simulink model "fc_KTH_lib"  (Simulink 4.00)
settings: Solver=FixedStepDiscrete  StartTime=0.0  StopTime=5  RelTol=1e-3
undefined symbols (not defined in the file or in its folder): cell_const_F, cell_const_g, cell_const_jo, cell_const_LHV_H2, cell_const_Mair, cell_const_MH, cell_const_MW, cell_const_R2, cell_const_Voc, fan_cool, fc_act, fc_blower_rec_H2, fc_blowera, fc_cell_const_eta1, fc_cell_const_eta_DCDC, fc_cell_const_etablow, fc_cell_const_etagen, fc_cell_const_etapump, fc_cell_const_ex, fc_cell_const_kw, fc_cell_const_Nrad, fc_cell_const_U, fc_cell_dim_A, fc_cell_dim_tm, fc_cell_press_a, fc_cell_press_amb, fc_cell_press_an, fc_cell_press_blowa, fc_cell_press_blowr, fc_cell_press_c, fc_cell_press_hum, fc_cell_press_hyd, fc_cell_stack_dpipe, fc_cell_stack_dpipefc, fc_cell_stack_drad, fc_cell_stack_Lpipe, fc_cell_stack_Lpipefc, fc_cell_stack_Lrad, fc_cell_stack_N, fc_cell_stack_Pel, fc_cell_stoich_RHah, fc_cell_stoich_RHch, fc_cell_stoich_RHo, fc_cell_stoich_vH, fc_cell_stoich_vO, fc_cell_stoich_XON, fc_cell_temp_ah, fc_cell_temp_amb, fc_cell_temp_cell, fc_cell_temp_ch, fc_cell_temp_cond, fc_cell_temp_cool, fc_cell_temp_evap, fc_cell_temp_rad, fc_cell_temp_ref, fc_compressor, fc_conda, fc_condc, fc_coolstack, fc_current ... (+10)
(part 1 of 2)
settings Model: LastModifiedBy=kharalds

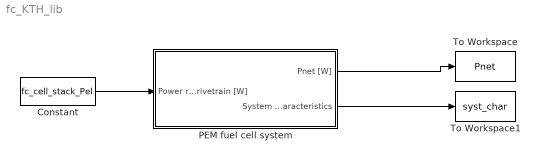
== system fc_KTH_lib ==
  Constant : Constant  Value=fc_cell_stack_Pel
  PEM fuel cell system : Subsystem
      settings: RTWFcnNameOpts=Auto  RTWFileNameOpts=Auto
  To Workspace : ToWorkspace  VariableName=Pnet  SampleTime=-1  SaveFormat=Array
  To Workspace1 : ToWorkspace  VariableName=syst_char  SampleTime=-1  SaveFormat=Array
  wires:
  Constant/1 -> PEM fuel cell system/1("Power request from drivetrain [W] ")
  PEM fuel cell system/1(Pnet [W]) -> To Workspace/1
  PEM fuel cell system/2(System characteristics) -> To Workspace1/1

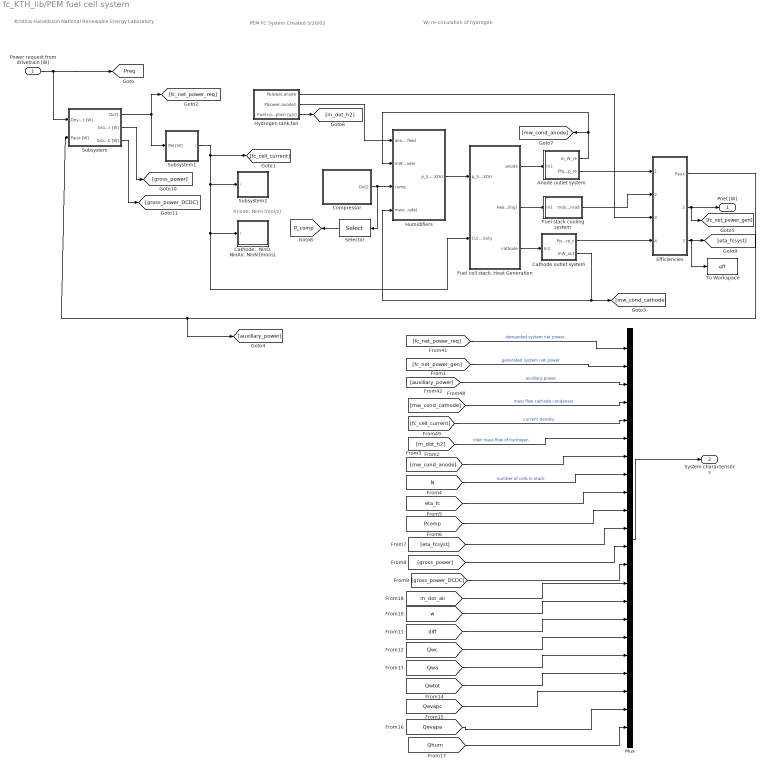
== system fc_KTH_lib/PEM fuel cell system ==
  note: Kristina Haraldsson
      | National Renewable Energy Laboratory
  note: PEM FC System
      | Created  3/20/02
  note: W/ re-circulation of hydrogen
  note: Anode: NinH [mol/s]
  "Power request from drivetrain [W] " : Inport  Port=1  LatchInput=off
  Anode outlet system : Subsystem
      settings: RTWFcnNameOpts=Auto  RTWFileNameOpts=Auto
  Cathode outlet system : Subsystem
      settings: RTWFcnNameOpts=Auto  RTWFileNameOpts=Auto
  "Cathode:  NinO, NinAir, NinN [mol/s]" : Subsystem
      settings: RTWFcnNameOpts=Auto  RTWFileNameOpts=Auto
  "Compressor " : Subsystem
      settings: RTWFcnNameOpts=Auto  RTWFileNameOpts=Auto
  Efficiencies : Subsystem
      settings: RTWFcnNameOpts=Auto  RTWFileNameOpts=Auto
  "Fuel cell stack, Heat Generation" : Subsystem
      settings: RTWFcnNameOpts=Auto  RTWFileNameOpts=Auto
  Fuel stack cooling system : Subsystem
      settings: RTWFcnNameOpts=Auto  RTWFileNameOpts=Auto
  Humidifiers : Subsystem
      settings: RTWFcnNameOpts=Auto  RTWFileNameOpts=Auto
  Hydrogen tank,fan : Subsystem
      settings: RTWFcnNameOpts=Auto  RTWFileNameOpts=Auto
  Mux : Mux  Inputs=22
  Selector : Selector  Orientation=left  InputType=Vector  ElementSrc=Internal  Elements=[4]  RowSrc=Internal  Rows=1  ColumnSrc=Internal  Columns=1  InputPortWidth=7
  Subsystem : Subsystem
      settings: RTWFcnNameOpts=Auto  RTWFileNameOpts=Auto
  Subsystem1 : Subsystem
      settings: RTWFcnNameOpts=Auto  RTWFileNameOpts=Auto
  Subsystem2 : Subsystem
      settings: RTWFcnNameOpts=Auto  RTWFileNameOpts=Auto
  To Workspace : ToWorkspace  VariableName=eff  SampleTime=-1  SaveFormat=Array
  Pnet [W] : Outport  Port=1
  System characteristics : Outport  Port=2
  tag scope: P_comp=global, Preq=global
  wires:
  Humidifiers/1("p_56 anode feed p_57 cathode feed Psat Psatah Psatch XWaI,  XWcI  XOcI ") -> "Fuel cell stack, Heat Generation"/1("p_56, NinH, p_57, NinAir, Psat,Psatah,PsatchXWaI, XWcI, XOcI")
  "Compressor "/1(Out2) -> Humidifiers/3(comp), Selector/1
  "Fuel cell stack, Heat Generation"/1(anode) -> Anode outlet system/1(In1)
  "Fuel cell stack, Heat Generation"/2(Heat_fc (fuel cell stack cooling)) -> Fuel stack cooling system/1(In1)
  Fuel stack cooling system/1(mdotW P_pump A Heat Qcool P_fanrad) -> Efficiencies/2(P_pump,cool P_fanrad)
  Anode outlet system/2(Pfan Ppump_re) -> Efficiencies/1("P_fan_,re, P_pump_re_a")
  Anode outlet system/1(m_W_re) -> Humidifiers/2(mW_out(anode)), [mw_cond_anode]
  "Fuel cell stack, Heat Generation"/3(cathode) -> Cathode outlet system/1(In1)
  Cathode outlet system/1(Ppump_re_c) -> Efficiencies/4(P_pump_re_c)
  Cathode outlet system/2(mW_out) -> Humidifiers/4(mwout(cathode)), [mw_cond_cathode]
  Hydrogen tank,fan/1(Pblower,anode) -> Efficiencies/3(P_fan,anode)
  Efficiencies/1(Paux) -> Subsystem/2(Paux [W]), [auxiliary_power]
  Subsystem/1(Out1) -> Subsystem1/1(Pel [W]), [fc_net_power_req]
  "Power request from drivetrain [W] "/1 -> Subsystem/1(Drivetrain Power Request [W]), [Preq]
  Subsystem1/1(i) -> Subsystem2/1(i), "Cathode:  NinO, NinAir, NinN [mol/s]"/1(i), "Fuel cell stack, Heat Generation"/2(Current density), [fc_cell_current]
  Hydrogen tank,fan/3(Fuel consumption [g/s]) -> [m_dot_h2]
  Hydrogen tank,fan/2(Pblower,anode1) -> Humidifiers/1(anode feed)
  [fc_net_power_req] -> Mux/1  "demanded system net power"
  [auxiliary_power] -> Mux/3  "auxiliary power"
  [mw_cond_cathode] -> Mux/4  "mass flow cathode condenser"
  [fc_cell_current] -> Mux/5  "current density"
  [fc_net_power_gen] -> Mux/2  "generated system net power"
  Mux/1 -> System characteristics/1
  [m_dot_h2] -> Mux/6  "inlet mass flow of hydrogen"
  [mw_cond_anode] -> Mux/7
  [N] -> Mux/8  "number of cells in stack"
  [eta_fc] -> Mux/9
  [Pcomp] -> Mux/10
  Selector/1 -> [P_comp]
  Subsystem/2(Gross power [W]) -> [gross_power]
  Efficiencies/2(Pnet [W]) -> Pnet [W]/1, [fc_net_power_gen]
  Efficiencies/3(eta_fcsyst) -> [eta_fcsyst], To Workspace/1
  Subsystem/3(Gross power incl. DCDC [W]) -> [gross_power_DCDC]
  [eta_fcsyst] -> Mux/11
  [gross_power] -> Mux/12
  [gross_power_DCDC] -> Mux/13
  [Qhum] -> Mux/22
  [Qevapa] -> Mux/21
  [Qevapc] -> Mux/20
  [Qwtot] -> Mux/19
  [Qwa] -> Mux/18
  [Qwc] -> Mux/17
  [diff] -> Mux/16
  [w] -> Mux/15
  [m_dot_air] -> Mux/14

== system fc_KTH_lib/PEM fuel cell system/Anode outlet system ==
  note: Anode outlet system
  In1 : Inport  Port=1  LatchInput=off
  Anode condenser : Subsystem
      settings: RTWFcnNameOpts=Auto  RTWFileNameOpts=Auto
  Mux : Mux  Inputs=2
  Mux1 : Mux  Inputs=2
  "Re-circulation: Blower_rec, pump" : Subsystem
      settings: RTWFcnNameOpts=Auto  RTWFileNameOpts=Auto
  Vent/Purge : Subsystem
      settings: RTWFcnNameOpts=Auto  RTWFileNameOpts=Auto
  m_W_re : Outport  Port=1
  Pfan Ppump_re : Outport  Port=2
  tag scope: NoutH=global
  wires:
  In1/1 -> Anode condenser/1(In1)
  Anode condenser/1(Out1) -> Vent/Purge/1(In1)
  Vent/Purge/1(Out1) -> "Re-circulation: Blower_rec, pump"/1(In1)
  "Re-circulation: Blower_rec, pump"/3(p_70) -> Mux/2
  "Re-circulation: Blower_rec, pump"/4(Pfan) -> Mux1/1
  "Re-circulation: Blower_rec, pump"/5(Ppump_re) -> Mux1/2
  Mux1/1 -> Pfan Ppump_re/1
  "Re-circulation: Blower_rec, pump"/1(m_W_re) -> m_W_re/1
  "Re-circulation: Blower_rec, pump"/2(NoutH_re) -> Mux/1
  Mux/1 -> [NoutH]

== system fc_KTH_lib/PEM fuel cell system/Cathode outlet system ==
  note: Cathode outlet system
  In1 : Inport  Port=1  LatchInput=off
  Cathode condenser : Subsystem
      settings: RTWFcnNameOpts=Auto  RTWFileNameOpts=Auto
  Pump (cathode) : Subsystem
      settings: RTWFcnNameOpts=Auto  RTWFileNameOpts=Auto
  Ppump_re_c : Outport  Port=1
  mW_out : Outport  Port=2
  wires:
  In1/1 -> Cathode condenser/1(In1)
  Pump (cathode)/1(Ppump_re_c) -> Ppump_re_c/1
  Cathode condenser/1(mw_out1) -> Pump (cathode)/1(In1)
  Pump (cathode)/2(mW_out) -> mW_out/1

== system fc_KTH_lib/PEM fuel cell system/Cathode:  NinO, NinAir, NinN [mol/s] ==
  note: Total cathode molar flow
  i : Inport  Port=1  LatchInput=off
  Constant : Constant  Value=fc_cell_stoich_vO
  Constant1 : Constant  Value=fc_cell_dim_A
  Constant2 : Constant  Value=fc_cell_stack_N
  Constant3 : Constant  Value=cell_const_F
  Constant4 : Constant  Value=4
  Constant5 : Constant  Value=fc_cell_stoich_XON
  Constant6 : Constant  Value=fc_cell_stoich_XON
  Constant7 : Constant  Value=1
  Constant8 : Constant  Value=cell_const_Mair
  Product : Product  Inputs=4  Multiplication=Element-wise(.*)  SaturateOnIntegerOverflow=on
  Product1 : Product  Inputs=*/  Multiplication=Element-wise(.*)  SaturateOnIntegerOverflow=on
  Product2 : Product  Inputs=2  Multiplication=Element-wise(.*)  SaturateOnIntegerOverflow=on
  Product3 : Product  Inputs=*/  Multiplication=Element-wise(.*)  SaturateOnIntegerOverflow=on
  Product4 : Product  Inputs=2  Multiplication=Element-wise(.*)  SaturateOnIntegerOverflow=on
  Product5 : Product  Inputs=2  Multiplication=Element-wise(.*)  SaturateOnIntegerOverflow=on
  Sum : Sum  Inputs=|+-  SaturateOnIntegerOverflow=on
  tag scope: NinAir=global, NinN=global, NinO=global, m_dot_air=global
  wires:
  Constant1/1 -> Product/3
  Constant/1 -> Product/2
  i/1 -> Product/1
  Constant2/1 -> Product/4
  Product/1 -> Product1/1
  Constant4/1 -> Product2/2
  Product2/1 -> Product1/2
  Product1/1 -> Product3/1, [NinO]
  Constant5/1 -> Product3/2
  Product3/1 -> Product4/1, Product5/1, [NinAir]
  Constant7/1 -> Sum/1
  Constant6/1 -> Sum/2
  Sum/1 -> Product4/2
  Product4/1 -> [NinN]
  Constant3/1 -> Product2/1
  Constant8/1 -> Product5/2
  Product5/1 -> [m_dot_air]

== system fc_KTH_lib/PEM fuel cell system/Compressor  ==
  note: Compressor
  Cathode pressure : Constant  Value=fc_cell_press_c
  "Initial value, 0.1 mole/s" : Memory  X0=0.1  InheritSampleTime=off
      settings: RTWStateStorageClass=Auto
  M_air [g/mol] : Constant  Value=cell_const_Mair
  Mass flow [g/s]  discharge pressure [bar(a)] CompOA1050 (Opcon) : Lookup  InputValues=[Qm_1050]  OutputValues=[p2_1050]
  Mass flow [g/s] Pcomp [W] CompOA1050 (Opcon) : Lookup  InputValues=[Qm_1050]  OutputValues=[Pcomp_1050]
  Mass flow [g/s] discharge temperature [C] CompOA1050 (Opcon)1 : Lookup  InputValues=[Qm_1050]  OutputValues=[T2_1050]
  Mux : Mux  Inputs=5
  Product : Product  Inputs=2  Multiplication=Element-wise(.*)  SaturateOnIntegerOverflow=on
  fc_compressor.m : MATLABFcn  MATLABFcn=fc_compressor(u,fc_cell_press_amb,fc_cell_temp_amb,fc_cell_const_eta1,fc_cell_const_etagen,fc_cell_stoich_RHo,fc_cell_press_hum,fc_cell_temp_evap,fc_cell_temp_cell,fc_cell_stack_Pel)  OutputDimensions=7  OutputSignalType=auto  Output1D=on
  Out2 : Outport  Port=1
  wires:
  M_air [g/mol]/1 -> Product/2
  Mux/1 -> fc_compressor.m/1
  fc_compressor.m/1 -> Out2/1
  Mass flow [g/s]  discharge pressure [bar(a)] CompOA1050 (Opcon)/1 -> Mux/2
  Mass flow [g/s] Pcomp [W] CompOA1050 (Opcon)/1 -> Mux/3
  [NinAir] -> "Initial value, 0.1 mole/s"/1
  "Initial value, 0.1 mole/s"/1 -> Mux/1, Product/1
  Product/1 -> Mass flow [g/s]  discharge pressure [bar(a)] CompOA1050 (Opcon)/1, Mass flow [g/s] Pcomp [W] CompOA1050 (Opcon)/1, Mass flow [g/s] discharge temperature [C] CompOA1050 (Opcon)1/1
  Mass flow [g/s] discharge temperature [C] CompOA1050 (Opcon)1/1 -> Mux/4
  Cathode pressure/1 -> Mux/5

== system fc_KTH_lib/PEM fuel cell system/Efficiencies ==
  note: Efficiencies
  "P_fan_,re, P_pump_re_a" : Inport  Port=1  LatchInput=off
  P_pump,cool P_fanrad : Inport  Port=2  LatchInput=off
  P_fan,anode : Inport  Port=3  LatchInput=off
  P_pump_re_c : Inport  Port=4  LatchInput=off
  Constant : Constant  Value=cell_const_LHV_H2
  Demux : Demux  Outputs=2  BusSelectionMode=off
  Demux1 : Demux  Outputs=2  BusSelectionMode=off
  Product : Product  Inputs=*/  Multiplication=Element-wise(.*)  SaturateOnIntegerOverflow=on
  Product1 : Product  Inputs=2  Multiplication=Element-wise(.*)  SaturateOnIntegerOverflow=on
  Selector1 : Selector  InputType=Vector  ElementSrc=Internal  Elements=[2 6]  RowSrc=Internal  Rows=1  ColumnSrc=Internal  Columns=1  InputPortWidth=6
  Sum{,1..6} (7 alike) : Sum  Inputs=|++  SaturateOnIntegerOverflow=on
  Sum7 : Sum  Inputs=|-+  SaturateOnIntegerOverflow=on
  Paux : Outport  Port=1
  Pnet [W] : Outport  Port=2
  eta_fcsyst : Outport  Port=3
  tag scope: Pcomp=global
  wires:
  P_pump,cool P_fanrad/1 -> Selector1/1
  [P_comp] -> Sum/1, [Pcomp]
  "P_fan_,re, P_pump_re_a"/1 -> Demux/1
  P_pump_re_c/1 -> Sum6/2
  P_fan,anode/1 -> Sum5/2
  Demux/1 -> Sum3/2
  Demux/2 -> Sum4/2
  [P_fancool] -> Sum/2
  Sum/1 -> Sum1/1
  Selector1/1 -> Demux1/1
  Demux1/1 -> Sum1/2
  Sum1/1 -> Sum2/1
  Demux1/2 -> Sum2/2
  Sum2/1 -> Sum3/1
  Sum3/1 -> Sum4/1
  Sum4/1 -> Sum5/1
  Sum5/1 -> Sum6/1
  Sum6/1 -> Sum7/1, Paux/1
  Sum7/1 -> Product/1, Pnet [W]/1
  [Preq] -> Sum7/2
  Constant/1 -> Product1/2
  [NinH] -> Product1/1
  Product1/1 -> Product/2
  Product/1 -> eta_fcsyst/1

== system fc_KTH_lib/PEM fuel cell system/Fuel cell stack, Heat Generation ==
  note: FCSystem_H2
      | /Fuel cell stack, Heat generation
  note: NinWa NinHa NoutWag NoutHa
      | NinWc NinO NinN NoutWcg NWlgen
      | NoutWcl NoutO NoutN Nout_condc Nout_conda
  "p_56, NinH, p_57, NinAir, Psat,Psatah,PsatchXWaI, XWcI, XOcI" : Inport  Port=1  LatchInput=off
  Current density : Inport  Port=2  LatchInput=off
  Constant1 : Constant  Value=cell_const_F
  Constant3 : Constant  Value=2
  Heat : Subsystem
      settings: RTWFcnNameOpts=Auto  RTWFileNameOpts=Auto
  J Water produced at cathode : Product  Inputs=/*  Multiplication=Element-wise(.*)  SaturateOnIntegerOverflow=on
  Mux1 : Mux  Inputs=5
  Product2 : Product  Inputs=2  Multiplication=Element-wise(.*)  SaturateOnIntegerOverflow=on
  fc_eqs : MATLABFcn  MATLABFcn=fc_eqs(u,fc_cell_dim_A,fc_cell_press_a,fc_cell_press_c,fc_cell_press_amb,fc_cell_stoich_RHo,cell_const_F,fc_cell_temp_cell,fc_cell_temp_ah,fc_cell_temp_ch,fc_cell_temp_amb,fc_cell_membrane_Mm,fc_cell_membrane_pdry,fc_cell_dim_tm,fc_cell_stoich_vO,fc_cell_stoich_vH,fc_cell_const_zw,fc_cell_stack_Pel,fc_cell_stack_N)  OutputDimensions=20  OutputSignalType=auto  Output1D=on
  flows : Selector  InputType=Vector  ElementSrc=Internal  Elements=[3 4 5 6 7 8 10 11 12 13 14 19 20]  RowSrc=Internal  Rows=1  ColumnSrc=Internal  Columns=1  InputPortWidth=20
  flows p_60 NoutWcg NoutWlgen NoutWcl NoutO NoutN Nout_condc : Selector  InputType=Vector  ElementSrc=Internal  Elements=[1 10 11 12 13 14 19]  RowSrc=Internal  Rows=1  ColumnSrc=Internal  Columns=1  InputPortWidth=20
  "p_61,NoutWag, NoutHa,NWAout,NoutWal" : Selector  InputType=Vector  ElementSrc=Internal  Elements=[2 5 6 16 17]  RowSrc=Internal  Rows=1  ColumnSrc=Internal  Columns=1  InputPortWidth=20
  anode : Outport  Port=1
  Heat_fc (fuel cell stack cooling) : Outport  Port=2
  cathode : Outport  Port=3
  tag scope: eta_fc=global
  wires:
  "p_56, NinH, p_57, NinAir, Psat,Psatah,PsatchXWaI, XWcI, XOcI"/1 -> Mux1/1
  "p_61,NoutWag, NoutHa,NWAout,NoutWal"/1 -> anode/1
  Mux1/1 -> fc_eqs/1
  fc_eqs/1 -> "p_61,NoutWag, NoutHa,NWAout,NoutWal"/1, flows/1, flows p_60 NoutWcg NoutWlgen NoutWcl NoutO NoutN Nout_condc/1
  flows/1 -> Heat/1(In1 NinWa NinHa NoutWag NoutHa NinWc NinO NinN NoutWcg NoutWcl NoutO NoutN Nout_condc Nout_conda)
  Heat/1(Heat_fc) -> Heat_fc (fuel cell stack cooling)/1
  [NinO] -> Mux1/2
  [NinN] -> Mux1/3
  [lambda] -> Mux1/4
  Current density/1 -> Heat/2(Current density [A/cm2]), J Water produced at cathode/2
  Heat/2(eta_fc) -> [eta_fc]
  flows p_60 NoutWcg NoutWlgen NoutWcl NoutO NoutN Nout_condc/1 -> cathode/1
  Constant1/1 -> Product2/1
  Constant3/1 -> Product2/2
  Product2/1 -> J Water produced at cathode/1
  J Water produced at cathode/1 -> Mux1/5

== system fc_KTH_lib/PEM fuel cell system/Fuel stack cooling system ==
  note: Fuel stack cooling system
  note: Cooling medium: air
  note: Cooling medium: water
  In1 : Inport  Port=1  LatchInput=off
  Display : Display
      settings: Format=short
  Display1 : Display
      settings: Format=short
  Pump_cool : Subsystem
      settings: RTWFcnNameOpts=Auto  RTWFileNameOpts=Auto
  Radiator : Subsystem
      settings: RTWFcnNameOpts=Auto  RTWFileNameOpts=Auto
  fan_cool : Subsystem
      settings: RTWFcnNameOpts=Auto  RTWFileNameOpts=Auto
  fuel stack cooling mass flows : Subsystem
      settings: RTWFcnNameOpts=Auto  RTWFileNameOpts=Auto
  mdotW P_pump A Heat Qcool P_fanrad : Outport  Port=1
  tag scope: P_fancool=global
  wires:
  In1/1 -> fuel stack cooling mass flows/1(In1)
  fuel stack cooling mass flows/1(Cooling water flow [kg/s] Cooling air flow [kg/s]) -> Pump_cool/1(In1), fan_cool/1(m_A,T1,Q,etafc)
  fan_cool/1(P_fancool) -> Display/1, [P_fancool]
  Pump_cool/1(Out1) -> Radiator/1(In1)
  Radiator/1(Out2) -> mdotW P_pump A Heat Qcool P_fanrad/1, Display1/1

== system fc_KTH_lib/PEM fuel cell system/Humidifiers ==
  note: Humidifiers
  anode feed : Inport  Port=1  LatchInput=off
  mW_out(anode) : Inport  Port=2  LatchInput=off
  comp : Inport  Port=3  LatchInput=off
  mwout(cathode) : Inport  Port=4  LatchInput=off
  Constant : Constant  Value=fc_cell_press_c
  Constant1 : Constant  Value=fc_cell_press_a
  Evapcooler : Subsystem
      settings: RTWFcnNameOpts=Auto  RTWFileNameOpts=Auto
  Memory : Memory  X0=[0.00058799]  InheritSampleTime=off
      settings: RTWStateStorageClass=Auto
  Memory (former value  1.280458) : Memory  X0=0.04  InheritSampleTime=off
      settings: RTWStateStorageClass=Auto
  Mux : Mux  Inputs=6
  Selector : Selector  InputType=Vector  ElementSrc=Internal  Elements=[1 2 3 4 5 6 7 8 9 10 ]  RowSrc=Internal  Rows=1  ColumnSrc=Internal  Columns=1  InputPortWidth=25
  "p_56 anode feed p_57 cathode feed Psat Psatah Psatch XWaI,  XWcI  XOcI " : Outport  Port=1
  wires:
  anode feed/1 -> Evapcooler/1(anode feed Thyd p NinHa Pfan)
  Selector/1 -> "p_56 anode feed p_57 cathode feed Psat Psatah Psatch XWaI,  XWcI  XOcI "/1
  mW_out(anode)/1 -> Memory/1
  Memory/1 -> Evapcooler/2(mW_out(anode))
  mwout(cathode)/1 -> Memory (former value  1.280458)/1
  Evapcooler/1(Out1) -> Selector/1
  [psat_air] -> Mux/1
  [psatah] -> Mux/2
  [psatch] -> Mux/3
  [XWaI] -> Mux/4
  [XWcI] -> Mux/5
  [XOcI] -> Mux/6
  Mux/1 -> Evapcooler/7("Psat,Psatah, PsatchXWaI,  XWcI, XOcI")
  Memory (former value  1.280458)/1 -> Evapcooler/3(mW_out(cathode))
  Constant/1 -> Evapcooler/4(Pc)
  Constant1/1 -> Evapcooler/5(Pa)
  comp/1 -> Evapcooler/6(comp)

== system fc_KTH_lib/PEM fuel cell system/Hydrogen tank,fan ==
  note: Hydrogen tank, blower
  note: Fuel consumption
      | [mol/s]
  Fcn : Fcn  Expr=u(4)
  MW hydrogen : Constant  Value=cell_const_MH
  Mux : Mux  Inputs=2
  NinH (initial fuel flow) [mol/s]  NinH (fuel cons.) [mol.s] : Selector  InputType=Vector  ElementSrc=Internal  Elements=[2]  RowSrc=Internal  Rows=1  ColumnSrc=Internal  Columns=1  InputPortWidth=2
  Product : Product  Inputs=2  Multiplication=Element-wise(.*)  SaturateOnIntegerOverflow=on
  Selector : Selector  InputType=Vector  ElementSrc=Internal  Elements=[1]  RowSrc=Internal  Rows=1  ColumnSrc=Internal  Columns=1  InputPortWidth=2
  Sum : Sum  Inputs=|+-  SaturateOnIntegerOverflow=on
  fc_blowera.m : MATLABFcn  MATLABFcn=fc_blowera(u,fc_cell_const_etablow,fc_cell_stack_dpipe,fc_cell_stack_Lpipe,cell_const_g,fc_cell_press_blowa,fc_cell_press_an,fc_cell_press_a,fc_cell_press_hum,fc_cell_temp_cell)  OutputDimensions=4  OutputSignalType=auto  Output1D=on
  Pblower,anode : Outport  Port=1
  Pblower,anode1 : Outport  Port=2
  Fuel consumption [g/s] : Outport  Port=3
  wires:
  fc_blowera.m/1 -> Fcn/1, Pblower,anode1/1
  Fcn/1 -> Pblower,anode/1
  Mux/1 -> NinH (initial fuel flow) [mol/s]  NinH (fuel cons.) [mol.s]/1
  [NinH] -> Sum/1, fc_blowera.m/1, Mux/1
  [NoutH] -> Selector/1
  MW hydrogen/1 -> Product/2
  NinH (initial fuel flow) [mol/s]  NinH (fuel cons.) [mol.s]/1 -> Product/1
  Product/1 -> Fuel consumption [g/s]/1
  Selector/1 -> Sum/2
  Sum/1 -> Mux/2

== system fc_KTH_lib/PEM fuel cell system/Subsystem ==
  note: Power Request
  Drivetrain Power Request [W] : Inport  Port=1  LatchInput=off
  Paux [W] : Inport  Port=2  LatchInput=off
  "Inverse of efficiency of DC/DC " : Constant  Orientation=up  Value=1/fc_cell_const_eta_DCDC
  Memory : Memory  X0=5000  InheritSampleTime=off
      settings: RTWStateStorageClass=Auto
  Preq=(Pel+Paux)/eta_DCDC : Product  Inputs=2  Multiplication=Element-wise(.*)  SaturateOnIntegerOverflow=on
  Sum1 : Sum  Inputs=|++  SaturateOnIntegerOverflow=on
  Out1 : Outport  Port=1
  Gross power [W] : Outport  Port=2
  Gross power incl. DCDC [W] : Outport  Port=3
  wires:
  Drivetrain Power Request [W]/1 -> Sum1/1
  Sum1/1 -> Gross power [W]/1, Preq=(Pel+Paux)/eta_DCDC/1
  "Inverse of efficiency of DC/DC "/1 -> Preq=(Pel+Paux)/eta_DCDC/2
  Preq=(Pel+Paux)/eta_DCDC/1 -> Out1/1, Gross power incl. DCDC [W]/1
  Paux [W]/1 -> Memory/1
  Memory/1 -> Sum1/2

== system fc_KTH_lib/PEM fuel cell system/Subsystem1 ==
  note: Calculation of number of cells, current density and cell voltage
  Pel [W] : Inport  Port=1  LatchInput=off
  Anode init : Subsystem
      settings: RTWFcnNameOpts=Auto  RTWFileNameOpts=Auto
  Cathode Overpotential : Subsystem
      settings: RTWFcnNameOpts=Auto  RTWFileNameOpts=Auto
  Cathode oxygen molar fraction : Subsystem
      settings: RTWFcnNameOpts=Auto  RTWFileNameOpts=Auto
  Cathode water molar fraction : Subsystem
      settings: RTWFcnNameOpts=Auto  RTWFileNameOpts=Auto
  Constant : Constant  Value=fc_cell_stack_N
  Demux : Demux  Outputs=3  BusSelectionMode=off
  Membrane conductivity : Subsystem
      settings: RTWFcnNameOpts=Auto  RTWFileNameOpts=Auto
  Membrane resistance : Subsystem
      settings: RTWFcnNameOpts=Auto  RTWFileNameOpts=Auto
  Mux : Mux  Inputs=4
  Saturation pressure  cathode humidifier : Subsystem
      settings: RTWFcnNameOpts=Auto  RTWFileNameOpts=Auto
  fc_current : MATLABFcn  MATLABFcn=fc_current(u,fc_cell_press_c,fc_cell_press_a,fc_cell_dim_tm,cell_const_F,cell_const_jo,cell_const_Voc,cell_const_R2,fc_cell_dim_A,fc_cell_temp_cell,fc_cell_temp_ah,fc_cell_temp_ch)  OutputDimensions=3  OutputSignalType=auto  Output1D=on
  i : Outport  Port=1
  tag scope: Ecell=global, N=global, XWaI=global, lambda=global, psatah=global
  wires:
  Membrane conductivity/1(Sigma) -> Membrane resistance/1(sigma)
  Anode init/1(lambda) -> Membrane conductivity/1(lambda), [lambda]
  Membrane resistance/1(Rm [ohm/cm2]) -> Mux/1
  Saturation pressure  cathode humidifier/1(psatch) -> Cathode water molar fraction/1(psatch [bar])
  Cathode water molar fraction/1(XWcI [-]) -> Cathode Overpotential/2(XWcI), Cathode oxygen molar fraction/1(XWcI [-]1)
  Cathode oxygen molar fraction/1(XOcI [-]) -> Cathode Overpotential/1(XOcI)
  Cathode Overpotential/1(Po) -> Mux/2
  Mux/1 -> fc_current/1
  Pel [W]/1 -> Mux/3
  fc_current/1 -> Demux/1
  Demux/3 -> [N]
  Constant/1 -> Mux/4
  Anode init/2(XWaI) -> [XWaI]
  Anode init/3(psatah) -> [psatah]
  Demux/2 -> [Ecell]
  Demux/1 -> i/1

== system fc_KTH_lib/PEM fuel cell system/Subsystem2 ==
  note: Total anode molar flow
  i : Inport  Port=1  LatchInput=off
  Constant : Constant  Value=fc_cell_stoich_vH
  Constant1 : Constant  Value=fc_cell_dim_A
  Constant2 : Constant  Value=fc_cell_stack_N
  Constant3 : Constant  Value=cell_const_F
  Constant4 : Constant  Value=2
  Constant5 : Constant  Value=cell_const_MH
  Display1 : Display
      settings: Format=short
  Product : Product  Inputs=4  Multiplication=Element-wise(.*)  SaturateOnIntegerOverflow=on
  Product1 : Product  Inputs=*/  Multiplication=Element-wise(.*)  SaturateOnIntegerOverflow=on
  Product2 : Product  Inputs=2  Multiplication=Element-wise(.*)  SaturateOnIntegerOverflow=on
  Product3 : Product  Inputs=2  Multiplication=Element-wise(.*)  SaturateOnIntegerOverflow=on
  To Workspace : ToWorkspace  VariableName=NinH  SampleTime=-1  SaveFormat=Array
  tag scope: NinH=global
  wires:
  Constant1/1 -> Product/3
  Constant/1 -> Product/2
  i/1 -> Product/1
  Constant2/1 -> Product/4
  Product/1 -> Product1/1
  Constant3/1 -> Product2/1
  Constant4/1 -> Product2/2
  Product2/1 -> Product1/2
  Product1/1 -> Product3/1, [NinH], To Workspace/1
  Constant5/1 -> Product3/2
  Product3/1 -> Display1/1

== system fc_KTH_lib/PEM fuel cell system/Anode outlet system/Anode condenser ==
  note: Anode outlet system/Anode condenser
  In1 : Inport  Port=1  LatchInput=off
  fc_conda : MATLABFcn  MATLABFcn=fc_conda(u,fc_cell_const_ex,fc_cell_temp_amb,fc_cell_temp_cond,fc_cell_temp_cell)  OutputDimensions=6  OutputSignalType=auto  Output1D=on
  Out1 : Outport  Port=1
  wires:
  In1/1 -> fc_conda/1
  fc_conda/1 -> Out1/1

== system fc_KTH_lib/PEM fuel cell system/Anode outlet system/Re-circulation: Blower_rec, pump ==
  note: Anode outlet system/Blower, pump
  In1 : Inport  Port=1  LatchInput=off
  Demux : Demux  Outputs=2  BusSelectionMode=off
  Demux1 : Demux  Outputs=3  BusSelectionMode=off
  Memory : Memory  X0=0.06848  InheritSampleTime=off
      settings: RTWStateStorageClass=Auto
  Memory1 : Memory  X0=2.59  InheritSampleTime=off
      settings: RTWStateStorageClass=Auto
  Selector1 : Selector  InputType=Vector  ElementSrc=Internal  Elements=[2 3 4]  RowSrc=Internal  Rows=1  ColumnSrc=Internal  Columns=1  InputPortWidth=5
  Selector2 : Selector  InputType=Vector  ElementSrc=Internal  Elements=[1 2]  RowSrc=Internal  Rows=1  ColumnSrc=Internal  Columns=1  InputPortWidth=5
  fc_blower_rec_H2 re-circulation of hydrogen : MATLABFcn  MATLABFcn=fc_blower_rec_H2(u,fc_cell_const_etablow,fc_cell_temp_cell,fc_cell_stack_dpipe,fc_cell_stack_Lpipe,fc_cell_press_blowr,cell_const_g,cell_const_MH)  OutputDimensions=5  OutputSignalType=auto  Output1D=on
  pump_re (re-circulation of water from the anode) : MATLABFcn  MATLABFcn=pump_re(u,fc_cell_temp_cond,cell_const_g,fc_cell_stack_dpipe,fc_cell_stack_Lpipe,fc_cell_const_etapump)  OutputDimensions=5  OutputSignalType=auto  Output1D=on
  m_W_re : Outport  Port=1
  NoutH_re : Outport  Port=2
  p_70 : Outport  Port=3
  Pfan : Outport  Port=4
  Ppump_re : Outport  Port=5
  wires:
  In1/1 -> pump_re (re-circulation of water from the anode)/1, fc_blower_rec_H2 re-circulation of hydrogen/1
  pump_re (re-circulation of water from the anode)/1 -> Selector2/1
  Selector2/1 -> Demux/1
  Demux/1 -> Ppump_re/1
  Demux/2 -> m_W_re/1
  Selector1/1 -> Demux1/1
  Demux1/2 -> Memory1/1
  fc_blower_rec_H2 re-circulation of hydrogen/1 -> Selector1/1
  Demux1/1 -> Memory/1
  Memory/1 -> NoutH_re/1
  Memory1/1 -> p_70/1
  Demux1/3 -> Pfan/1

== system fc_KTH_lib/PEM fuel cell system/Anode outlet system/Vent/Purge ==
  note: Anode outlet system/Purge
  In1 : Inport  Port=1  LatchInput=off
  vent : MATLABFcn  MATLABFcn=vent(u,fc_cell_const_ex)  OutputDimensions=10  OutputSignalType=auto  Output1D=on
  Out1 : Outport  Port=1
  wires:
  In1/1 -> vent/1
  vent/1 -> Out1/1

== system fc_KTH_lib/PEM fuel cell system/Cathode outlet system/Cathode condenser ==
  note: Cathode outlet system/Cathode condenser
  In1 : Inport  Port=1  LatchInput=off
  Mux : Mux  Inputs=2
  Saturation temperature : Subsystem
      settings: RTWFcnNameOpts=Auto  RTWFileNameOpts=Auto
  Selector : Selector  InputType=Vector  ElementSrc=Internal  Elements=[1]  RowSrc=Internal  Rows=1  ColumnSrc=Internal  Columns=1  InputPortWidth=7
  fc_condc : MATLABFcn  MATLABFcn=fc_condc(u,fc_cell_temp_amb,fc_cell_temp_cond,fc_cell_temp_ch,fc_cell_temp_cell)  OutputDimensions=7  OutputSignalType=auto  Output1D=on
  mw_out : Selector  InputType=Vector  ElementSrc=Internal  Elements=[4]  RowSrc=Internal  Rows=1  ColumnSrc=Internal  Columns=1  InputPortWidth=7
  mw_out1 : Outport  Port=1
  wires:
  In1/1 -> Mux/1, Selector/1
  fc_condc/1 -> mw_out/1
  mw_out/1 -> mw_out1/1
  Mux/1 -> fc_condc/1
  Saturation temperature/1(Temp [K]) -> Mux/2
  Selector/1 -> Saturation temperature/1(pressure [bar])

== system fc_KTH_lib/PEM fuel cell system/Cathode outlet system/Pump (cathode) ==
  note: Cathode outlet system/Pump (cathode)
  note: mw_out
      | condensed water from
      |  the cathode
  In1 : Inport  Port=1  LatchInput=off
  Selector : Selector  InputType=Vector  ElementSrc=Internal  Elements=[2]  RowSrc=Internal  Rows=1  ColumnSrc=Internal  Columns=1  InputPortWidth=2
  Selector1 : Selector  InputType=Vector  ElementSrc=Internal  Elements=[1]  RowSrc=Internal  Rows=1  ColumnSrc=Internal  Columns=1  InputPortWidth=2
  pump2 (re-circulation of water from the cathode) : MATLABFcn  MATLABFcn=pump2(u,fc_cell_temp_cond,cell_const_g,fc_cell_stack_dpipe,fc_cell_stack_Lpipe,fc_cell_const_etapump)  OutputDimensions=2  OutputSignalType=auto  Output1D=on
  Ppump_re_c : Outport  Port=1
  mW_out : Outport  Port=2
  wires:
  In1/1 -> pump2 (re-circulation of water from the cathode)/1
  pump2 (re-circulation of water from the cathode)/1 -> Selector/1, Selector1/1
  Selector/1 -> Ppump_re_c/1
  Selector1/1 -> mW_out/1

== system fc_KTH_lib/PEM fuel cell system/Fuel cell stack, Heat Generation/Heat ==
  note: Heat & efficiency of fuel cell stack
  In1 NinWa NinHa NoutWag NoutHa NinWc NinO NinN NoutWcg NoutWcl NoutO NoutN Nout_condc Nout_conda : Inport  Port=1  LatchInput=off
  Current density [A/cm2] : Inport  Port=2  LatchInput=off
  Demux : Demux  Outputs=13  BusSelectionMode=off
  Fuel cell efficiency : Subsystem
      settings: RTWFcnNameOpts=Auto  RTWFileNameOpts=Auto
  Heat generation [W] : Subsystem
      settings: RTWFcnNameOpts=Auto  RTWFileNameOpts=Auto
  Latent heat [W] : Subsystem
      settings: RTWFcnNameOpts=Auto  RTWFileNameOpts=Auto
  Reaction heat [W] : Subsystem
      settings: RTWFcnNameOpts=Auto  RTWFileNameOpts=Auto
  Sensible heat [W] : Subsystem
      settings: RTWFcnNameOpts=Auto  RTWFileNameOpts=Auto
  Sum : Sum  Inputs=|++  SaturateOnIntegerOverflow=on
  Heat_fc : Outport  Port=1
  eta_fc : Outport  Port=2
  wires:
  In1 NinWa NinHa NoutWag NoutHa NinWc NinO NinN NoutWcg NoutWcl NoutO NoutN Nout_condc Nout_conda/1 -> Demux/1
  Demux/1 -> Sensible heat [W]/1(NinWa)
  Demux/2 -> Sensible heat [W]/2(NinHa)
  Demux/3 -> Sensible heat [W]/3(NoutWag)
  Demux/4 -> Sensible heat [W]/4(NoutHa)
  Demux/5 -> Sensible heat [W]/5(NinWc)
  Demux/6 -> Sensible heat [W]/6(NinO)
  Demux/7 -> Sensible heat [W]/7(NInN)
  Demux/8 -> Sensible heat [W]/8(NoutWcg)
  Demux/9 -> Sensible heat [W]/9(NoutWcl)
  Demux/10 -> Sensible heat [W]/10(NoutO)
  Demux/11 -> Sensible heat [W]/11(NoutN)
  Demux/12 -> Sum/1
  Demux/13 -> Sum/2
  Sum/1 -> Latent heat [W]/1(NWcond)
  Current density [A/cm2]/1 -> Reaction heat [W]/1(Current density)
  [Ecell] -> Reaction heat [W]/2(Ecell), Fuel cell efficiency/2(Ecell)
  Sensible heat [W]/1(sensin) -> Heat generation [W]/1(sensin)
  Sensible heat [W]/2(sensout) -> Heat generation [W]/2(sensout)
  Latent heat [W]/1(latheat [W]) -> Heat generation [W]/3(latheat)
  Reaction heat [W]/1(reaheat [W]) -> Heat generation [W]/4(reaheat)
  Heat generation [W]/1(Heat_fc) -> Heat_fc/1
  Reaction heat [W]/2(Hr [J/mol]) -> Fuel cell efficiency/1(Hr)
  Fuel cell efficiency/1(eta_fc) -> eta_fc/1

== system fc_KTH_lib/PEM fuel cell system/Fuel stack cooling system/Pump_cool ==
  note: Fuel stack cooling system/Pumpcool
  In1 : Inport  Port=1  LatchInput=off
  pump_cool.m : MATLABFcn  MATLABFcn=pump_cool(u,fc_cell_temp_cool,cell_const_g,fc_cell_stack_dpipefc,fc_cell_stack_Lpipefc,fc_cell_const_etapump,fc_cell_temp_cell,fc_cell_stack_Lpipe,fc_cell_stack_dpipe,fc_cell_stack_N)  OutputDimensions=6  OutputSignalType=auto  Output1D=on
  Out1 : Outport  Port=1
  wires:
  In1/1 -> pump_cool.m/1
  pump_cool.m/1 -> Out1/1

== system fc_KTH_lib/PEM fuel cell system/Fuel stack cooling system/Radiator ==
  note: Cooling system/Radiator
  In1 : Inport  Port=1  LatchInput=off
  radiator.m : MATLABFcn  MATLABFcn=radiator(u,fc_cell_temp_amb,fc_cell_temp_rad,fc_cell_const_U,fc_cell_temp_cool,fc_cell_const_kw,fc_cell_stack_dpipe,fc_cell_stack_Lpipe,fc_cell_const_etablow,fc_cell_temp_cell,cell_const_g,fc_cell_stack_drad,fc_cell_stack_Lrad,fc_cell_const_Nrad)  OutputDimensions=6  OutputSignalType=auto  Output1D=on
  Out2 : Outport  Port=1
  wires:
  radiator.m/1 -> Out2/1
  In1/1 -> radiator.m/1

== system fc_KTH_lib/PEM fuel cell system/Fuel stack cooling system/fan_cool ==
  note: Cooling system/Fan_cool
  m_A,T1,Q,etafc : Inport  Port=1  LatchInput=off
  Selector : Selector  InputType=Vector  ElementSrc=Internal  Elements=[2]  RowSrc=Internal  Rows=1  ColumnSrc=Internal  Columns=1  InputPortWidth=4
  fan_cool.m : MATLABFcn  MATLABFcn=fan_cool(u,fc_cell_temp_cool,fc_cell_temp_cell,cell_const_g,fc_cell_stack_dpipefc,fc_cell_stack_Lpipefc,fc_cell_const_etablow,fc_cell_press_amb,fc_cell_press_blowr)  OutputDimensions=4  OutputSignalType=auto  Output1D=on
  P_fancool : Outport  Port=1
  wires:
  m_A,T1,Q,etafc/1 -> fan_cool.m/1
  fan_cool.m/1 -> Selector/1
  Selector/1 -> P_fancool/1

== system fc_KTH_lib/PEM fuel cell system/Fuel stack cooling system/fuel stack cooling mass flows ==
  note: Fuel stack cooling system/Fuel stack cooling, mass flows
  In1 : Inport  Port=1  LatchInput=off
  fc_coolstack.m : MATLABFcn  MATLABFcn=fc_coolstack(u,fc_cell_temp_cool,fc_cell_temp_amb,fc_cell_temp_cell)  OutputDimensions=4  OutputSignalType=auto  Output1D=on
  Cooling water flow [kg/s] Cooling air flow [kg/s] : Outport  Port=1
  wires:
  In1/1 -> fc_coolstack.m/1
  fc_coolstack.m/1 -> Cooling water flow [kg/s] Cooling air flow [kg/s]/1

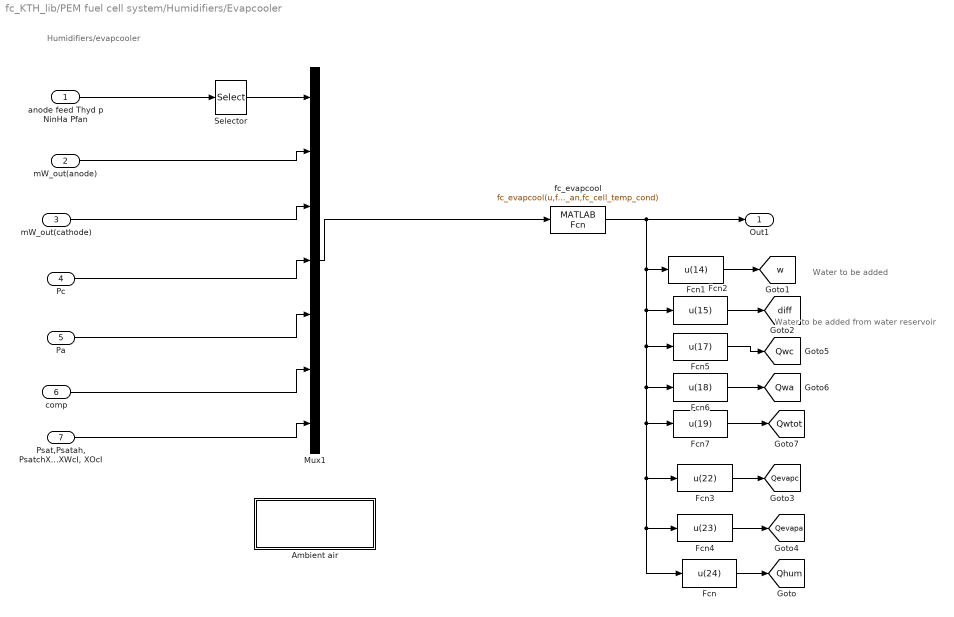
== system fc_KTH_lib/PEM fuel cell system/Humidifiers/Evapcooler ==
  note: Humidifiers/evapcooler
  note: Water to be added
  note: Water to be added
      | from water reservoir
  anode feed Thyd p NinHa Pfan : Inport  Port=1  LatchInput=off
  mW_out(anode) : Inport  Port=2  LatchInput=off
  mW_out(cathode) : Inport  Port=3  LatchInput=off
  Pc : Inport  Port=4  LatchInput=off
  Pa : Inport  Port=5  LatchInput=off
  comp : Inport  Port=6  LatchInput=off
  "Psat,Psatah, PsatchXWaI,  XWcI, XOcI" : Inport  Port=7  LatchInput=off
  Ambient air : Subsystem
      settings: RTWFcnNameOpts=Auto  RTWFileNameOpts=Auto
  Fcn : Fcn  Expr=u(24)
  Fcn1 : Fcn  Expr=u(14)
  Fcn2 : Fcn  Expr=u(15)
  Fcn3 : Fcn  Expr=u(22)
  Fcn4 : Fcn  Expr=u(23)
  Fcn5 : Fcn  Expr=u(17)
  Fcn6 : Fcn  Expr=u(18)
  Fcn7 : Fcn  Expr=u(19)
  Mux1 : Mux  Inputs=7
  Selector : Selector  InputType=Vector  ElementSrc=Internal  Elements=[1 2 3]  RowSrc=Internal  Rows=1  ColumnSrc=Internal  Columns=1  InputPortWidth=4
  fc_evapcool : MATLABFcn  MATLABFcn=fc_evapcool(u,fc_cell_temp_cell,fc_cell_temp_evap,fc_cell_press_hum,fc_cell_press_hyd,fc_cell_stoich_RHah,fc_cell_stoich_RHch,fc_cell_press_an,fc_cell_temp_cond)  OutputDimensions=25  OutputSignalType=auto  Output1D=on
  Out1 : Outport  Port=1
  tag scope: Qevapa=global, Qevapc=global, Qhum=global, Qwa=global, Qwc=global, Qwtot=global, diff=global, w=global
  wires:
  mW_out(anode)/1 -> Mux1/2
  Pa/1 -> Mux1/5
  Pc/1 -> Mux1/4
  mW_out(cathode)/1 -> Mux1/3
  Mux1/1 -> fc_evapcool/1
  fc_evapcool/1 -> Out1/1, Fcn1/1, Fcn2/1, Fcn5/1, Fcn6/1, Fcn3/1, Fcn/1, Fcn4/1, Fcn7/1
  anode feed Thyd p NinHa Pfan/1 -> Selector/1
  Selector/1 -> Mux1/1
  comp/1 -> Mux1/6
  "Psat,Psatah, PsatchXWaI,  XWcI, XOcI"/1 -> Mux1/7
  Fcn/1 -> [Qhum]
  Fcn1/1 -> [w]
  Fcn2/1 -> [diff]
  Fcn3/1 -> [Qevapc]
  Fcn4/1 -> [Qevapa]
  Fcn5/1 -> [Qwc]
  Fcn6/1 -> [Qwa]
  Fcn7/1 -> [Qwtot]

== system fc_KTH_lib/PEM fuel cell system/Subsystem1/Anode init ==
  note: Anode
      | Saturation pressure, water fraction, activity, lambda
  Anode water molar fraction : Subsystem
      settings: RTWFcnNameOpts=Auto  RTWFileNameOpts=Auto
  Saturation pressure  anode humidifier : Subsystem
      settings: RTWFcnNameOpts=Auto  RTWFileNameOpts=Auto
  Subsystem2 : Subsystem
      settings: RTWFcnNameOpts=Auto  RTWFileNameOpts=Auto
  fc_act.m : MATLABFcn  MATLABFcn=fc_act(u)  OutputDimensions=1  OutputSignalType=auto  Output1D=on
  lambda : Outport  Port=1
  XWaI : Outport  Port=2
  psatah : Outport  Port=3
  wires:
  Saturation pressure  anode humidifier/1(psatah) -> Anode water molar fraction/1(psatah [bar]), Subsystem2/2(psatah [bar]), psatah/1
  Anode water molar fraction/1(XWaI [-]) -> Subsystem2/1(XWaI [-]), XWaI/1
  Subsystem2/1(a) -> fc_act.m/1
  fc_act.m/1 -> lambda/1

== system fc_KTH_lib/PEM fuel cell system/Subsystem1/Cathode Overpotential ==
  note: Cathode overpotential
  XOcI : Inport  Port=1  LatchInput=off
  XWcI : Inport  Port=2  LatchInput=off
  Cathode pressure : Constant  Value=fc_cell_press_c
  Constant1 : Constant  Value=1
  Product : Product  Inputs=*/  Multiplication=Element-wise(.*)  SaturateOnIntegerOverflow=on
  Product1 : Product  Inputs=2  Multiplication=Element-wise(.*)  SaturateOnIntegerOverflow=on
  Sum : Sum  Inputs=|+-  SaturateOnIntegerOverflow=on
  Po : Outport  Port=1
  wires:
  Constant1/1 -> Sum/1
  XWcI/1 -> Sum/2
  XOcI/1 -> Product/1
  Sum/1 -> Product/2
  Product/1 -> Product1/1
  Cathode pressure/1 -> Product1/2
  Product1/1 -> Po/1

== system fc_KTH_lib/PEM fuel cell system/Subsystem1/Cathode oxygen molar fraction ==
  note: Oxygen molar fraction in the cathode inlet stream
  XWcI [-]1 : Inport  Port=1  LatchInput=off
  0.21 : Constant  Value=fc_cell_stoich_XON
  Constant1 : Constant  Value=1
  Product2 : Product  Inputs=2  Multiplication=Element-wise(.*)  SaturateOnIntegerOverflow=on
  Sum : Sum  Inputs=|+-  SaturateOnIntegerOverflow=on
  XOcI [-] : Outport  Port=1
  tag scope: XOcI=global
  wires:
  Product2/1 -> XOcI [-]/1, [XOcI]
  Constant1/1 -> Sum/1
  XWcI [-]1/1 -> Sum/2
  Sum/1 -> Product2/1
  0.21/1 -> Product2/2

== system fc_KTH_lib/PEM fuel cell system/Subsystem1/Cathode water molar fraction ==
  note: Water molar fraction in the cathode inlet stream
  psatch [bar] : Inport  Port=1  LatchInput=off
  Cathode pressure : Constant  Value=fc_cell_press_c
  Constant4 : Constant  Value=100
  Product : Product  Inputs=*/  Multiplication=Element-wise(.*)  SaturateOnIntegerOverflow=on
  Product1 : Product  Inputs=*/  Multiplication=Element-wise(.*)  SaturateOnIntegerOverflow=on
  Product2 : Product  Inputs=2  Multiplication=Element-wise(.*)  SaturateOnIntegerOverflow=on
  Relative humidity cathode : Constant  Value=fc_cell_stoich_RHch
  XWcI [-] : Outport  Port=1
  tag scope: XWcI=global
  wires:
  Relative humidity cathode/1 -> Product1/1
  Constant4/1 -> Product1/2
  psatch [bar]/1 -> Product/1
  Cathode pressure/1 -> Product/2
  Product1/1 -> Product2/1
  Product/1 -> Product2/2
  Product2/1 -> XWcI [-]/1, [XWcI]

== system fc_KTH_lib/PEM fuel cell system/Subsystem1/Membrane conductivity ==
  note: Membrane conductivity
      | Nafion 117
  lambda : Inport  Port=1  LatchInput=off
  Constant : Constant  Value=0.005139
  Constant1 : Constant  Value=0.00326
  Constant2 : Constant  Value=303
  Constant3 : Constant  Value=273
  Constant4 : Constant  Value=1268
  Constant5 : Constant  Value=fc_cell_temp_cell
  Constant6 : Constant  Value=1
  Constant8 : Constant  Value=1
  Math Function : Math  Operator=exp  OutputSignalType=auto
  Product : Product  Inputs=2  Multiplication=Element-wise(.*)  SaturateOnIntegerOverflow=on
  Product1 : Product  Inputs=2  Multiplication=Element-wise(.*)  SaturateOnIntegerOverflow=on
  Product2 : Product  Inputs=*/  Multiplication=Element-wise(.*)  SaturateOnIntegerOverflow=on
  Product3 : Product  Inputs=*/  Multiplication=Element-wise(.*)  SaturateOnIntegerOverflow=on
  Product4 : Product  Inputs=2  Multiplication=Element-wise(.*)  SaturateOnIntegerOverflow=on
  Sum : Sum  Inputs=|+-  SaturateOnIntegerOverflow=on
  Sum1 : Sum  Inputs=|++  SaturateOnIntegerOverflow=on
  Sum2 : Sum  Inputs=|+-  SaturateOnIntegerOverflow=on
  Sigma : Outport  Port=1
  wires:
  lambda/1 -> Product/1
  Constant/1 -> Product/2
  Product/1 -> Sum/1
  Constant1/1 -> Sum/2
  Sum/1 -> Product1/1
  Constant6/1 -> Product2/1
  Constant2/1 -> Product2/2
  Constant8/1 -> Product3/1
  Sum1/1 -> Product3/2
  Constant3/1 -> Sum1/1
  Constant5/1 -> Sum1/2
  Product2/1 -> Sum2/1
  Product3/1 -> Sum2/2
  Constant4/1 -> Product4/1
  Sum2/1 -> Product4/2
  Product4/1 -> Math Function/1
  Math Function/1 -> Product1/2
  Product1/1 -> Sigma/1

== system fc_KTH_lib/PEM fuel cell system/Subsystem1/Membrane resistance ==
  note: Membrane resistance [ohm/cm2]
  sigma : Inport  Port=1  LatchInput=off
  Constant : Constant  Value=fc_cell_dim_tm
  Product : Product  Inputs=*/  Multiplication=Element-wise(.*)  SaturateOnIntegerOverflow=on
  Rm [ohm/cm2] : Outport  Port=1
  wires:
  Constant/1 -> Product/1
  sigma/1 -> Product/2
  Product/1 -> Rm [ohm/cm2]/1

== system fc_KTH_lib/PEM fuel cell system/Subsystem1/Saturation pressure  cathode humidifier ==
  note: Saturation pressure of water in the cathode humidifier
      | NOTE: [bar]
      | Data from "Anlaggnings- och apparatteknik", Westerlund, T., Abo Akademi, Finland, 1998
  Cathode humidifier temperature [C] : Constant  Value=fc_cell_temp_ch
  Cathode humidifier temperature [C]1 : Constant  Value=fc_cell_temp_ch
  Constant : Constant  Value=11.78
  Constant1 : Constant  Value=99.64
  Constant2 : Constant  Value=230
  Math Function : Math  Operator=exp  OutputSignalType=auto
  Product : Product  Inputs=*/  Multiplication=Element-wise(.*)  SaturateOnIntegerOverflow=on
  Product1 : Product  Inputs=2  Multiplication=Element-wise(.*)  SaturateOnIntegerOverflow=on
  Sum : Sum  Inputs=|+-  SaturateOnIntegerOverflow=on
  Sum1 : Sum  Inputs=|++  SaturateOnIntegerOverflow=on
  psatch : Outport  Port=1
  tag scope: psatch=global
  wires:
  Cathode humidifier temperature [C]/1 -> Sum/1
  Constant1/1 -> Sum/2
  Cathode humidifier temperature [C]1/1 -> Sum1/1
  Constant2/1 -> Sum1/2
  Sum/1 -> Product/1
  Sum1/1 -> Product/2
  Constant/1 -> Product1/2
  Product/1 -> Product1/1
  Product1/1 -> Math Function/1
  Math Function/1 -> psatch/1, [psatch]

== system fc_KTH_lib/PEM fuel cell system/Cathode outlet system/Cathode condenser/Saturation temperature ==
  note: Saturation temperature [K]
      | --------------------------------------------
      |  Data from L. Wester, 1998
      |  valid: 273.16<=Tsat<600 K and 0.000611<=p<12.33 MPa
      |
      | A=42.6776;
      | B=-3892.70;
      | C=-9.48654;
      |
      | T=A+B/(log(p)+C);
  pressure [bar] : Inport  Port=1  LatchInput=off
  A : Constant  Value=42.6776
  B : Constant  Value=-3892.70
  C : Constant  Value=-9.48654
  Constant : Constant  Value=100000
  Math Function : Math  Operator=log  OutputSignalType=auto
  Product : Product  Inputs=*/  Multiplication=Element-wise(.*)  SaturateOnIntegerOverflow=on
  Sum : Sum  Inputs=|++  SaturateOnIntegerOverflow=on
  Sum1 : Sum  Inputs=|++  SaturateOnIntegerOverflow=on
  "[bar] to [MPa]" : Product  Inputs=*/  Multiplication=Element-wise(.*)  SaturateOnIntegerOverflow=on
  Temp [K] : Outport  Port=1
  wires:
  pressure [bar]/1 -> "[bar] to [MPa]"/1
  Constant/1 -> "[bar] to [MPa]"/2
  A/1 -> Sum/1
  B/1 -> Product/1
  C/1 -> Sum1/2
  Sum1/1 -> Temp [K]/1
  Product/1 -> Sum/2
  Sum/1 -> Sum1/1
  "[bar] to [MPa]"/1 -> Math Function/1
  Math Function/1 -> Product/2

== system fc_KTH_lib/PEM fuel cell system/Fuel cell stack, Heat Generation/Heat/Fuel cell efficiency ==
  note: Fuel cell efficiency
      | -----------------------------
      | eta_fc=(-2*F*Ecell)/Hr;
  Hr : Inport  Port=1  LatchInput=off
  Ecell : Inport  Port=2  LatchInput=off
  Constant : Constant  Value=cell_const_F
  Constant1 : Constant  Value=2
  Gain : Gain  Gain=-1  Multiplication=Element-wise(K.*u)  SaturateOnIntegerOverflow=on
  Product : Product  Inputs=/*  Multiplication=Element-wise(.*)  SaturateOnIntegerOverflow=on
  Product2 : Product  Inputs=3  Multiplication=Element-wise(.*)  SaturateOnIntegerOverflow=on
  eta_fc : Outport  Port=1
  wires:
  Ecell/1 -> Gain/1
  Gain/1 -> Product2/1
  Constant/1 -> Product2/2
  Constant1/1 -> Product2/3
  Hr/1 -> Product/1
  Product2/1 -> Product/2
  Product/1 -> eta_fc/1

== system fc_KTH_lib/PEM fuel cell system/Fuel cell stack, Heat Generation/Heat/Heat generation [W] ==
  note: Heat generation [W]
      | --------------------------------
      | Heat=reaheat+ latheat+ sensin-sensout
  sensin : Inport  Port=1  LatchInput=off
  sensout : Inport  Port=2  LatchInput=off
  latheat : Inport  Port=3  LatchInput=off
  reaheat : Inport  Port=4  LatchInput=off
  Sum : Sum  Inputs=|+-  SaturateOnIntegerOverflow=on
  Sum1 : Sum  Inputs=|++  SaturateOnIntegerOverflow=on
  Sum2 : Sum  Inputs=|++  SaturateOnIntegerOverflow=on
  Heat_fc : Outport  Port=1
  wires:
  sensin/1 -> Sum/1
  sensout/1 -> Sum/2
  Sum/1 -> Sum1/1
  latheat/1 -> Sum1/2
  Sum1/1 -> Sum2/1
  reaheat/1 -> Sum2/2
  Sum2/1 -> Heat_fc/1

== system fc_KTH_lib/PEM fuel cell system/Fuel cell stack, Heat Generation/Heat/Latent heat [W] ==
  note: Latent heat
      | ---------------------
      | latheat= Hcond*NWcond
  NWcond : Inport  Port=1  LatchInput=off
  Heat of condensation : Subsystem
      settings: RTWFcnNameOpts=Auto  RTWFileNameOpts=Auto
  Product : Product  Inputs=2  Multiplication=Element-wise(.*)  SaturateOnIntegerOverflow=on
  latheat [W] : Outport  Port=1
  wires:
  NWcond/1 -> Product/1
  Heat of condensation/1(Hcond [J/mol]) -> Product/2
  Product/1 -> latheat [W]/1

== system fc_KTH_lib/PEM fuel cell system/Fuel cell stack, Heat Generation/Heat/Reaction heat [W] ==
  note: Reaction heat [W]
      | -------------------------------
      | NHion = 2*i*A/(2*F);
      | reaheat = (-Hr - 2*F*Ecell)*NHion;
  Current density : Inport  Port=1  LatchInput=off
  Ecell : Inport  Port=2  LatchInput=off
  Constant : Constant  Value=cell_const_F
  Constant1 : Constant  Value=cell_const_F
  Constant2 : Constant  Value=fc_cell_dim_A
  Constant3 : Constant  Value=2
  Gain : Gain  Gain=-1  Multiplication=Element-wise(K.*u)  SaturateOnIntegerOverflow=on
  Heat of reaction : Subsystem
      settings: RTWFcnNameOpts=Auto  RTWFileNameOpts=Auto
  NHion : Product  Inputs=*/  Multiplication=Element-wise(.*)  SaturateOnIntegerOverflow=on
  Product : Product  Inputs=2  Multiplication=Element-wise(.*)  SaturateOnIntegerOverflow=on
  Product1 : Product  Inputs=2  Multiplication=Element-wise(.*)  SaturateOnIntegerOverflow=on
  Product2 : Product  Inputs=3  Multiplication=Element-wise(.*)  SaturateOnIntegerOverflow=on
  Sum : Sum  Inputs=|+-  SaturateOnIntegerOverflow=on
  reaheat [W] : Outport  Port=1
  Hr [J/mol] : Outport  Port=2
  wires:
  Current density/1 -> Product1/1
  Constant2/1 -> Product1/2
  Product1/1 -> NHion/1
  Constant/1 -> NHion/2
  NHion/1 -> Product/1
  Product/1 -> reaheat [W]/1
  Heat of reaction/1(Hr [J/mol]) -> Gain/1, Hr [J/mol]/1
  Ecell/1 -> Product2/1
  Constant1/1 -> Product2/2
  Constant3/1 -> Product2/3
  Gain/1 -> Sum/1
  Product2/1 -> Sum/2
  Sum/1 -> Product/2

== system fc_KTH_lib/PEM fuel cell system/Fuel cell stack, Heat Generation/Heat/Sensible heat [W] ==
  note: Sensible heat in and out [W]
      | ------------------------------------------------
      | sensouta = NoutWag*HWgout + NoutHa*HHout+NoutWal*HWl;
      | sensoutc = NoutWcg*HWgout + NoutWcl*HWl + NoutO*HOout + NoutN*HNout;
      |
      | sensin = sensina + sensinc;
      | sensout = sensouta + sensoutc;
  NinWa : Inport  Port=1  LatchInput=off
  NinHa : Inport  Port=2  LatchInput=off
  NoutWag : Inport  Port=3  LatchInput=off
  NoutHa : Inport  Port=4  LatchInput=off
  NinWc : Inport  Port=5  LatchInput=off
  NinO : Inport  Port=6  LatchInput=off
  NInN : Inport  Port=7  LatchInput=off
  NoutWcg : Inport  Port=8  LatchInput=off
  NoutWcl : Inport  Port=9  LatchInput=off
  NoutO : Inport  Port=10  LatchInput=off
  NoutN : Inport  Port=11  LatchInput=off
  "Sensible heat in " : Subsystem
      settings: RTWFcnNameOpts=Auto  RTWFileNameOpts=Auto
  Sensible heat out : Subsystem
      settings: RTWFcnNameOpts=Auto  RTWFileNameOpts=Auto
  Sum : Sum  Inputs=|++  SaturateOnIntegerOverflow=on
  Sum1 : Sum  Inputs=|++  SaturateOnIntegerOverflow=on
  sensin : Outport  Port=1
  sensout : Outport  Port=2
  wires:
  "Sensible heat in "/1(sensina [W]) -> Sum/1
  NinWa/1 -> "Sensible heat in "/1(NinWa)
  NinHa/1 -> "Sensible heat in "/2(NinHa)
  NinWc/1 -> "Sensible heat in "/3(NinWc)
  NinO/1 -> "Sensible heat in "/4(NinO)
  NInN/1 -> "Sensible heat in "/5(NinN)
  "Sensible heat in "/2(sensinc [W]) -> Sum/2
  NoutWag/1 -> Sensible heat out/1(NoutWag)
  NoutHa/1 -> Sensible heat out/2(NoutHa)
  NoutWcg/1 -> Sensible heat out/3(NoutWcg)
  NoutO/1 -> Sensible heat out/4(NoutO)
  NoutN/1 -> Sensible heat out/5(NoutN)
  NoutWcl/1 -> Sensible heat out/6(NoutWcl)
  Sum/1 -> sensin/1
  Sensible heat out/1(sensouta [W]) -> Sum1/1
  Sensible heat out/2(sensoutc [W]) -> Sum1/2
  Sum1/1 -> sensout/1

== system fc_KTH_lib/PEM fuel cell system/Humidifiers/Evapcooler/Ambient air ==
  note: Ambient air
  Humidity in air : Subsystem
      settings: RTWFcnNameOpts=Auto  RTWFileNameOpts=Auto
  Saturation pressure : Subsystem
      settings: RTWFcnNameOpts=Auto  RTWFileNameOpts=Auto
  wires:
  Saturation pressure/1(psat_air) -> Humidity in air/1(psat_air)

== system fc_KTH_lib/PEM fuel cell system/Subsystem1/Anode init/Anode water molar fraction ==
  note: Water molar fraction in the anode inlet stream
  psatah [bar] : Inport  Port=1  LatchInput=off
  Anode pressure : Constant  Value=fc_cell_press_a
  Constant4 : Constant  Value=100
  Product : Product  Inputs=*/  Multiplication=Element-wise(.*)  SaturateOnIntegerOverflow=on
  Product1 : Product  Inputs=*/  Multiplication=Element-wise(.*)  SaturateOnIntegerOverflow=on
  Product2 : Product  Inputs=2  Multiplication=Element-wise(.*)  SaturateOnIntegerOverflow=on
  Relative humidity anode : Constant  Value=fc_cell_stoich_RHah
  XWaI [-] : Outport  Port=1
  wires:
  Relative humidity anode/1 -> Product1/1
  Constant4/1 -> Product1/2
  psatah [bar]/1 -> Product/1
  Anode pressure/1 -> Product/2
  Product1/1 -> Product2/1
  Product/1 -> Product2/2
  Product2/1 -> XWaI [-]/1
